simulink model "trajectories_sim"  (R2023b)
settings: Solver=FixedStepAuto  StartTime=0.0  StopTime=t_sim  FixedStep=t_int  MaxStep=t_int  RelTol=1e-3
values from neighbouring files (symbols this model uses):
  abe = j/10    [step2_trajectories_sim_script.m]
libraries: shared3dof x1
settings Model: Creator=aless  LastModifiedBy=aless

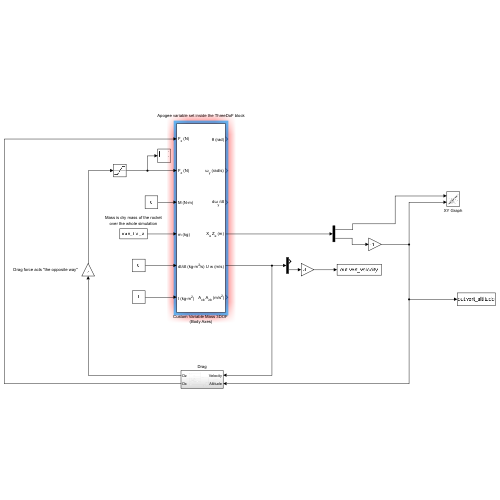
[thumbnail: Simulink's stored preview of the top-level diagram]
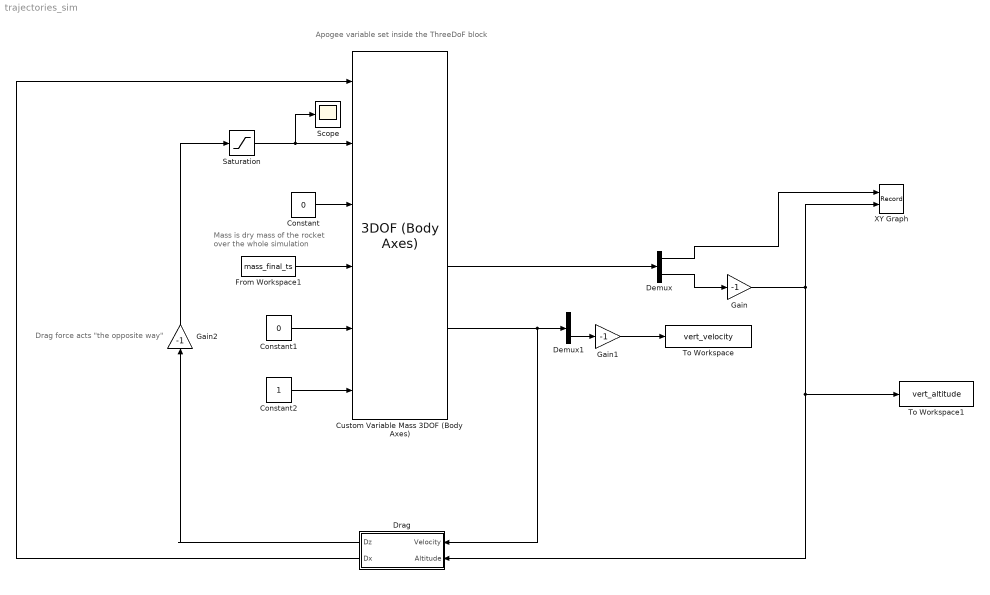
== system trajectories_sim ==
  note: Apogee variable set inside the ThreeDoF block
  note: Drag force acts "the opposite way"
  note: Mass is dry mass of the rocket
      | over the whole simulation
  Constant : Constant  Value=0
  Constant1 : Constant  Value=0
  Constant2 : Constant
  Custom Variable Mass 3DOF (Body Axes) : shared3dof/3DOF (Body Axes)  units=Metric (MKS)  mtype=Custom Variable  v_ini=0  theta_ini=launch_attitude  alpha_ini=0  pos_ini=init_pos  q_ini=0  mass=1.0  mass_e=0.5  mass_f=3.0  Iyy=1.0  Iyy_e=0.5  Iyy_f=3.0  g_in=Internal  g=9.81  vre_flag=off  abi_flag=off  aMode=0  vel_statename=''  theta_statename=''  pos_statename=''  q_statename=''  mass_statename=''
  Demux : Demux  Outputs=2
  Demux1 : Demux  Outputs=2
  Drag : Subsystem
  From Workspace1 : FromWorkspace  VariableName=mass_final_ts  OutputAfterFinalValue=Holding final value
  Gain : Gain  Gain=-1
  Gain1 : Gain  Gain=-1
  Gain2 : Gain  Gain=-1
  Saturation : Saturate  UpperLimit=1e5  LowerLimit=-1e5
  Scope : Scope
  To Workspace : ToWorkspace  VariableName=vert_velocity  SaveFormat=Timeseries  SampleTime=-1
  To Workspace1 : ToWorkspace  VariableName=vert_altitude  SaveFormat=Timeseries  SampleTime=-1
  XY Graph : Record  FileSettingsInternal="{\"entries\":[{\"content\":{\"excelSettings\":{\"content\":{},\"type\":\"Streamout.ExcelSettings\"}},\"type\":\"Streamout.FileSettingStorage\",\"uuid\":\"\"}],\"packageUris\":[\"http:\\/\\/schema.mathworks.com\\/mf0\\/streamout_blocks\\/R2020a\"],\"version\":\"1.0\"}"  Layout=[1 1]  SignalsInternal="{\"entries\":[{\"content\":{\"signals\":[{\"content\":{\"blockPath\":[],\"dimensions\":[1],\"domain\":\"\",\"lineColor\":\"#a2142f\",\"plots\":[ 1 ],\"port\":1,\"sid\":[\"\"],\"signalID\":1,\"signalName\":\"Demux:1\"},\"type\":\"RecordBlkView.Signal\",\"uuid\":\"\"},{\"content\":{\"blockPath\":[],\"dimensions\":[1],\"domain\":\"\",\"lineColor\":\"#139fff\",\"plots\":[ 1 ],\"port\":2,\"sid\":[\"\"],\"signalID\":2,\"signalName\":\"Gain\"},\"type\":\"RecordBlkView.Signal\",\"uuid\":\"\"}]},\"type\":\"RecordBlkView.InputSignals\",\"uuid\":\"\"}],\"packageUris\":[\"http:\\/\\/schema.mathworks.com\\/mf0\\/streamout_blocks\\/R2020a\"],\"version\":\"1.0\"}"  VisualizationBindings="{\"xyplotplugin\":{\"info\":[{\"series\":[{\"bindingParametersList\":[{\"parameter\":\"X-Axis\",\"signalID\":1,\"signalName\":\"Demux:1\"},{\"parameter\":\"Y-Axis\",\"signalID\":2,\"signalName\":\"Gain\"}],\"seriesID\":0}],\"subplotID\":1}]}}"  CompatibilityTag=XY  st=-1
  wires:
  From Workspace1/1 -> Custom Variable Mass 3DOF (Body Axes)/4
  Constant1/1 -> Custom Variable Mass 3DOF (Body Axes)/5
  Gain/1 -> XY Graph/2, To Workspace1/1, Drag/2(Altitude)
  Drag/2(Dx) -> Custom Variable Mass 3DOF (Body Axes)/1
  Custom Variable Mass 3DOF (Body Axes)/4 -> Demux/1
  Constant2/1 -> Custom Variable Mass 3DOF (Body Axes)/6
  Constant/1 -> Custom Variable Mass 3DOF (Body Axes)/3
  Demux/1 -> XY Graph/1
  Custom Variable Mass 3DOF (Body Axes)/5 -> Demux1/1, Drag/1(Velocity)
  Demux/2 -> Gain/1
  Drag/1(Dz) -> Gain2/1
  Demux1/2 -> Gain1/1
  Gain1/1 -> To Workspace/1
  Gain2/1 -> Saturation/1
  Saturation/1 -> Custom Variable Mass 3DOF (Body Axes)/2, Scope/1

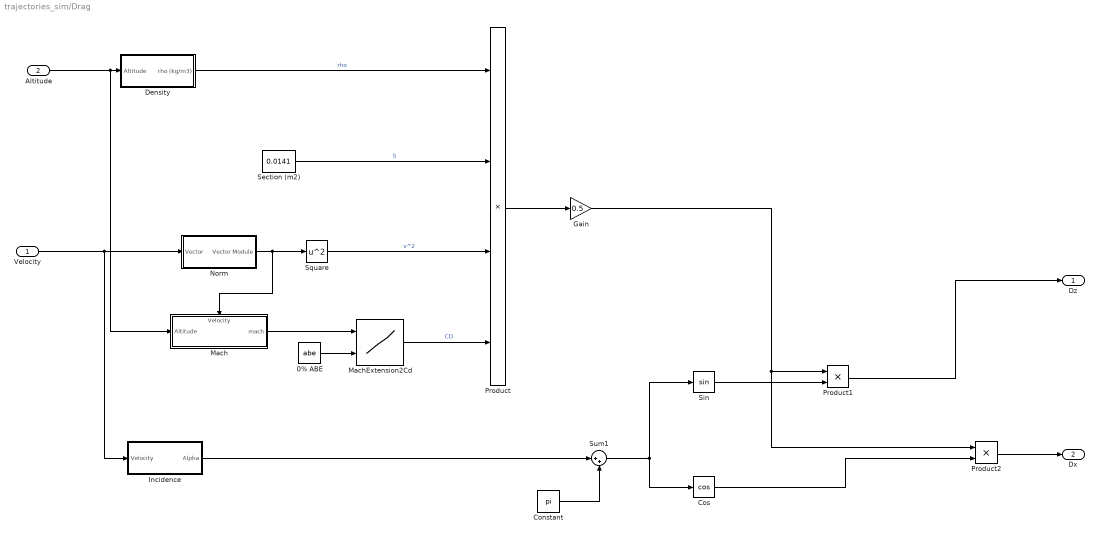
== system trajectories_sim/Drag ==
  Velocity : Inport
  Altitude : Inport  Port=2
  0% ABE : Constant  Value=abe
  Constant : Constant  Value=pi
  Cos : Trigonometry  Operator=cos
  Density : Subsystem
  Gain : Gain  Gain=0.5
  Incidence : Subsystem
  Mach : Subsystem
      settings: PortSchema="{\"entries\":[{\"content\":{\"sides\":[{\"content\":{\"connectorIds\":[\"In1\"]},\"type\":\"ConnectorPlacement.EquallySpacedRectSide\",\"uuid\":\"3d39723d-d359-4481-8e57-a1560243478f\"},{\"content\":{\"connectorIds\":[\"Out1\"],\"side\":\"RIGHT\"},\"type\":\"ConnectorPlacement.EquallySpacedRectSide\",\"uuid\":\"25d074cf-118b-4153-b466-e753361fe918\"},{\"content\":{\"connectorIds\":[\"In2\"],\"side\":\"TOP\"},\"type\":\"ConnectorPlacement.EquallySpacedRectSide\",\"uuid\":\"b814a212-e79e-4e83-ade8-85d301fd4927\"}]},\"type\":\"ConnectorPlacement.EquallySpacedConnector\",\"uuid\":\"c89f41df-1f7d-46ca-b296-160aff391222\"}],\"packageUris\":[\"http://schema.mathworks.com/mf0/Connector/R2020b\"],\"version\":\"1.0\"}"
  MachExtension2Cd : Lookup_n-D  DataSpecification=Lookup table object  LookupTableObject=surfaceBlockParameters1  BreakpointsForDimension1=[1:3]  BreakpointsForDimension2=[1:3]  ExtrapMethod=Clip  InternalRulePriority=Speed  RndMeth=Simplest
      settings: AttributesFormatString=Extrapolation=%<ExtrapMethod>  InputPortMap=u0,u1
  Norm : Subsystem
  Product : Product  Inputs=4
  Product1 : Product
  Product2 : Product
  Section (m2) : Constant  Value=0.0141
  Sin : Trigonometry
  Square : Math  Operator=square
  Sum1 : Sum  Inputs=|++
  Dz : Outport
  Dx : Outport  Port=2
  wires:
  Velocity/1 -> Incidence/1(Velocity), Norm/1(Vector)
  Altitude/1 -> Mach/1(Altitude), Density/1(Altitude)
  Incidence/1(Alpha) -> Sum1/1
  Norm/1(Vector Module) -> Square/1, Mach/2(Velocity)
  Density/1(rho (kg/m3)) -> Product/1  "rho"
  Section (m2)/1 -> Product/2  "S"
  Square/1 -> Product/3  "v^2"
  Product/1 -> Gain/1
  MachExtension2Cd/1 -> Product/4  "CD"
  Constant/1 -> Sum1/2
  Sum1/1 -> Sin/1, Cos/1
  Sin/1 -> Product1/2
  Gain/1 -> Product2/1, Product1/1
  Cos/1 -> Product2/2
  Product2/1 -> Dx/1
  Product1/1 -> Dz/1
  Mach/1(mach) -> MachExtension2Cd/1
  0% ABE/1 -> MachExtension2Cd/2

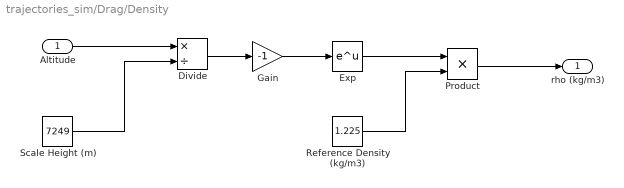
== system trajectories_sim/Drag/Density ==
  Altitude : Inport
  Divide : Product  Inputs=*/
  Exp : Math
  Gain : Gain  Gain=-1
  Product : Product
  Reference Density (kg/m3) : Constant  Value=1.225
  Scale Height (m) : Constant  Value=7249
  rho (kg/m3) : Outport
  wires:
  Altitude/1 -> Divide/1
  Scale Height (m)/1 -> Divide/2
  Divide/1 -> Gain/1
  Gain/1 -> Exp/1
  Exp/1 -> Product/1
  Reference Density (kg/m3)/1 -> Product/2
  Product/1 -> rho (kg/m3)/1

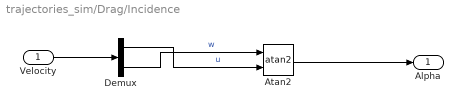
== system trajectories_sim/Drag/Incidence ==
  Velocity : Inport
  Atan2 : Trigonometry  Operator=atan2
  Demux : Demux  Outputs=2
  Alpha : Outport
  wires:
  Velocity/1 -> Demux/1
  Demux/2 -> Atan2/1  "w"
  Demux/1 -> Atan2/2  "u"
  Atan2/1 -> Alpha/1

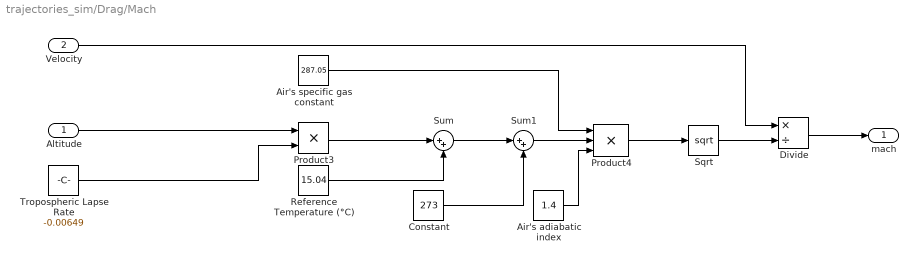
== system trajectories_sim/Drag/Mach ==
  Altitude : Inport
  Velocity : Inport  Port=2
  Air's adiabatic index : Constant  Value=1.4
  Air's specific gas constant : Constant  Value=287.05
  Constant : Constant  Value=273
  Divide : Product  Inputs=*/
  Product3 : Product
  Product4 : Product  Inputs=3
  Reference Temperature (°C) : Constant  Value=15.04
  Sqrt : Sqrt
  Sum : Sum  Inputs=|++
  Sum1 : Sum  Inputs=|++
  Tropospheric Lapse Rate : Constant  Value=-0.00649
  mach : Outport
  wires:
  Product4/1 -> Sqrt/1
  Product3/1 -> Sum/1
  Air's adiabatic index/1 -> Product4/3
  Tropospheric Lapse Rate/1 -> Product3/2
  Air's specific gas constant/1 -> Product4/1
  Sum/1 -> Sum1/1
  Reference Temperature (°C)/1 -> Sum/2
  Altitude/1 -> Product3/1
  Velocity/1 -> Divide/1
  Divide/1 -> mach/1
  Constant/1 -> Sum1/2
  Sum1/1 -> Product4/2
  Sqrt/1 -> Divide/2

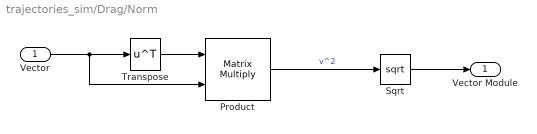
== system trajectories_sim/Drag/Norm ==
  Vector : Inport
  Product : Product  Multiplication=Matrix(*)
  Sqrt : Sqrt
  Transpose : Math  Operator=transpose
  Vector Module : Outport
  wires:
  Vector/1 -> Product/2, Transpose/1
  Product/1 -> Sqrt/1  "v^2"
  Sqrt/1 -> Vector Module/1
  Transpose/1 -> Product/1
